simulink model "PID_sim_test_coa"  (R2020b)
settings: Solver=VariableStepAuto  StartTime=0.0  StopTime=5  RelTol=1e-3
libraries: simulink x1
settings Model: Creator=ja  LastModifiedBy=ja

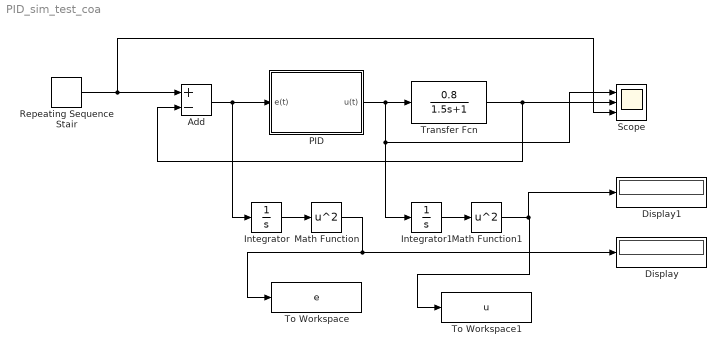
== system PID_sim_test_coa ==
  Add : Sum  Inputs=+-
  Display : Display
  Display1 : Display
  Integrator : Integrator
  Integrator1 : Integrator
  Math Function : Math  Operator=square  SaturateOnIntegerOverflow=on
  Math Function1 : Math  Operator=square  SaturateOnIntegerOverflow=on
  PID : Subsystem  mask{Kp=49.6735, Ki=1.8713, Kd=0.2095}
  Repeating Sequence Stair : simulink/Sources/Repeating Sequence Stair  OutValues=[1 2 4 3 1].'  tsamp=1  OutMin=[]  OutMax=[]  OutDataTypeStr=double  OutputDataTypeScalingMode=double  OutDataType=fixdt(0,8)  ConRadixGroup=Best Precision: Vector-wise  OutScaling=2^-12
  Scope : Scope  NumInputPorts=3
  To Workspace : ToWorkspace  VariableName=e  SaveFormat=Structure With Time  SampleTime=-1
  To Workspace1 : ToWorkspace  VariableName=u  SaveFormat=Structure With Time  SampleTime=-1
  Transfer Fcn : TransferFcn  Numerator=[0.8]  Denominator=[1.5 1]
  wires:
  Repeating Sequence Stair/1 -> Scope/3, Add/1
  Transfer Fcn/1 -> Add/2, Scope/2
  PID/1(u(t)) -> Integrator1/1, Scope/1, Transfer Fcn/1
  Add/1 -> Integrator/1, PID/1(e(t))
  Integrator/1 -> Math Function/1
  Integrator1/1 -> Math Function1/1
  Math Function1/1 -> Display1/1, To Workspace1/1
  Math Function/1 -> Display/1, To Workspace/1

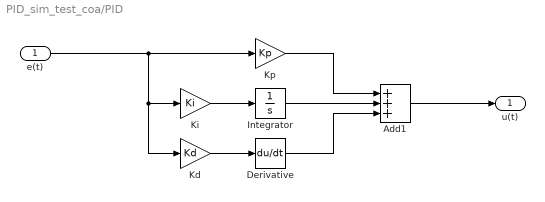
== system PID_sim_test_coa/PID ==
  e(t) : Inport
  Add1 : Sum  Inputs=+++
  Derivative : Derivative
  Integrator : Integrator
  Kd : Gain  Gain=Kd
  Ki : Gain  Gain=Ki
  Kp : Gain  Gain=Kp
  u(t) : Outport
  wires:
  Ki/1 -> Integrator/1
  Derivative/1 -> Add1/3
  Add1/1 -> u(t)/1
  Kd/1 -> Derivative/1
  e(t)/1 -> Kd/1, Ki/1, Kp/1
  Integrator/1 -> Add1/2
  Kp/1 -> Add1/1
